simulink model "Satellite_Attitude_Control_Scenario_B_final"  (R2026a)
settings: Solver=ode23s  StopTime=100  MaxStep=1e-2
libraries: simulink x3, slpidlib x3, matrix_library x1
settings Model: Creator=sreecharan  LastModifiedBy=sreecharan

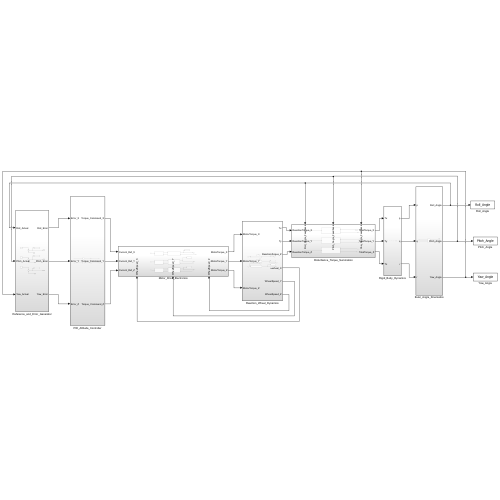
[thumbnail: Simulink's stored preview of the top-level diagram]
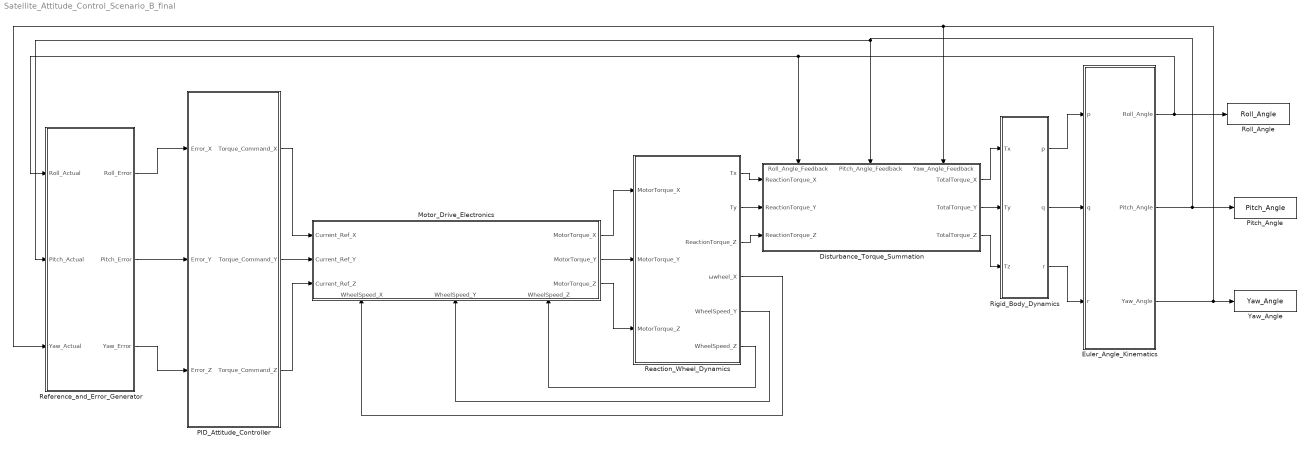
== system Satellite_Attitude_Control_Scenario_B_final ==
  Disturbance_Torque_Summation : Subsystem
      settings: PortSchema="{\"entries\":[{\"content\":{\"sides\":[{\"content\":{\"connectorIds\":[\"In1\",\"In2\",\"In3\"]},\"type\":\"ConnectorPlacement.EquallySpacedRectSide\",\"uuid\":\"7e4f6ff0-8d01-44c4-971d-6abc5d35a402\"},{\"content\":{\"connectorIds\":[\"Out1\",\"Out2\",\"Out3\"],\"side\":\"RIGHT\"},\"type\":\"ConnectorPlacement.EquallySpacedRectSide\",\"uuid\":\"cb81acf3-b383-4a7c-a155-f8d32ed2ffd6\"},{\"content\":{\"connectorIds\":[\"In4\",\"In5\",\"In6\"],\"side\":\"TOP\"},\"type\":\"ConnectorPlacement.EquallySpacedRectSide\",\"uuid\":\"aada53d5-02c2-40d2-a0ce-2f4cf8738fbf\"}]},\"type\":\"ConnectorPlacement.EquallySpacedConnector\",\"uuid\":\"ed5a9e7d-2126-4c89-bcb0-b7263c99b71f\"}],\"packageUris\":[\"http://schema.mathworks.com/mf0/Connector/R2020b\"],\"version\":\"1.0\"}"
  Euler_Angle_Kinematics : Subsystem
  Motor_Drive_Electronics : Subsystem
      settings: PortSchema="{\"entries\":[{\"content\":{\"sides\":[{\"content\":{\"connectorIds\":[\"In1\",\"In2\",\"In3\"]},\"type\":\"ConnectorPlacement.EquallySpacedRectSide\",\"uuid\":\"7e4f6ff0-8d01-44c4-971d-6abc5d35a402\"},{\"content\":{\"connectorIds\":[\"Out1\",\"Out2\",\"Out3\"],\"side\":\"RIGHT\"},\"type\":\"ConnectorPlacement.EquallySpacedRectSide\",\"uuid\":\"cb81acf3-b383-4a7c-a155-f8d32ed2ffd6\"},{\"content\":{\"side\":\"TOP\"},\"type\":\"ConnectorPlacement.EquallySpacedRectSide\",\"uuid\":\"aada53d5-02c2-40d2-a0ce-2f4cf8738fbf\"},{\"content\":{\"connectorIds\":[\"In4\",\"In5\",\"In6\"],\"side\":\"BOTTOM\"},\"type\":\"ConnectorPlacement.EquallySpacedRectSide\",\"uuid\":\"90859111-4cc3-4175-9d43-5206a627f844\"}]},\"type\":\"ConnectorPlacement.EquallySpacedConnector\",\"uuid\":\"ed5a9e7d-2126-4c89-bcb0-b7263c99b71f\"}],\"packageUris\":[\"http://schema.mathworks.com/mf0/Connector/R2020b\"],\"version\":\"1.0\"}"
  PID_Attitude_Controller : Subsystem
  Pitch_Angle : ToWorkspace  VariableName=Pitch_Angle  SampleTime=-1
  Reaction_Wheel_Dynamics : Subsystem
  Reference_and_Error_Generator : Subsystem
  Rigid_Body_Dynamics : Subsystem
  Roll_Angle : ToWorkspace  VariableName=Roll_Angle  SampleTime=-1
  Yaw_Angle : ToWorkspace  VariableName=Yaw_Angle  SampleTime=-1
  wires:
  Disturbance_Torque_Summation/1(TotalTorque_X) -> Rigid_Body_Dynamics/1(Tx)
  Disturbance_Torque_Summation/2(TotalTorque_Y) -> Rigid_Body_Dynamics/2(Ty)
  Disturbance_Torque_Summation/3(TotalTorque_Z) -> Rigid_Body_Dynamics/3(Tz)
  Motor_Drive_Electronics/2(MotorTorque_Y) -> Reaction_Wheel_Dynamics/2(MotorTorque_Y)
  Reaction_Wheel_Dynamics/1(Tx) -> Disturbance_Torque_Summation/1(ReactionTorque_X)
  Reaction_Wheel_Dynamics/2(Ty) -> Disturbance_Torque_Summation/2(ReactionTorque_Y)
  Reaction_Wheel_Dynamics/3(ReactionTorque_Z) -> Disturbance_Torque_Summation/3(ReactionTorque_Z)
  Reaction_Wheel_Dynamics/4(ωwheel_X) -> Motor_Drive_Electronics/4(WheelSpeed_X)
  Reaction_Wheel_Dynamics/5(WheelSpeed_Y) -> Motor_Drive_Electronics/5(WheelSpeed_Y)
  Reaction_Wheel_Dynamics/6(WheelSpeed_Z) -> Motor_Drive_Electronics/6(WheelSpeed_Z)
  Reference_and_Error_Generator/1(Roll_Error) -> PID_Attitude_Controller/1(Error_X)
  Reference_and_Error_Generator/2(Pitch_Error) -> PID_Attitude_Controller/2(Error_Y)
  Reference_and_Error_Generator/3(Yaw_Error) -> PID_Attitude_Controller/3(Error_Z)
  PID_Attitude_Controller/1(Torque_Command_X) -> Motor_Drive_Electronics/1(Current_Ref_X)
  PID_Attitude_Controller/2(Torque_Command_Y) -> Motor_Drive_Electronics/2(Current_Ref_Y)
  PID_Attitude_Controller/3(Torque_Command_Z) -> Motor_Drive_Electronics/3(Current_Ref_Z)
  Rigid_Body_Dynamics/1(p) -> Euler_Angle_Kinematics/1(p)
  Rigid_Body_Dynamics/2(q) -> Euler_Angle_Kinematics/2(q)
  Rigid_Body_Dynamics/3(r) -> Euler_Angle_Kinematics/3(r)
  Euler_Angle_Kinematics/1(Roll_Angle) -> Disturbance_Torque_Summation/4(Roll_Angle_Feedback), Reference_and_Error_Generator/1(Roll_Actual), Roll_Angle/1
  Euler_Angle_Kinematics/2(Pitch_Angle) -> Reference_and_Error_Generator/2(Pitch_Actual), Disturbance_Torque_Summation/5(Pitch_Angle_Feedback), Pitch_Angle/1
  Euler_Angle_Kinematics/3(Yaw_Angle) -> Disturbance_Torque_Summation/6(Yaw_Angle_Feedback), Reference_and_Error_Generator/3(Yaw_Actual), Yaw_Angle/1
  Motor_Drive_Electronics/3(MotorTorque_Z) -> Reaction_Wheel_Dynamics/3(MotorTorque_Z)
  Motor_Drive_Electronics/1(MotorTorque_X) -> Reaction_Wheel_Dynamics/1(MotorTorque_X)

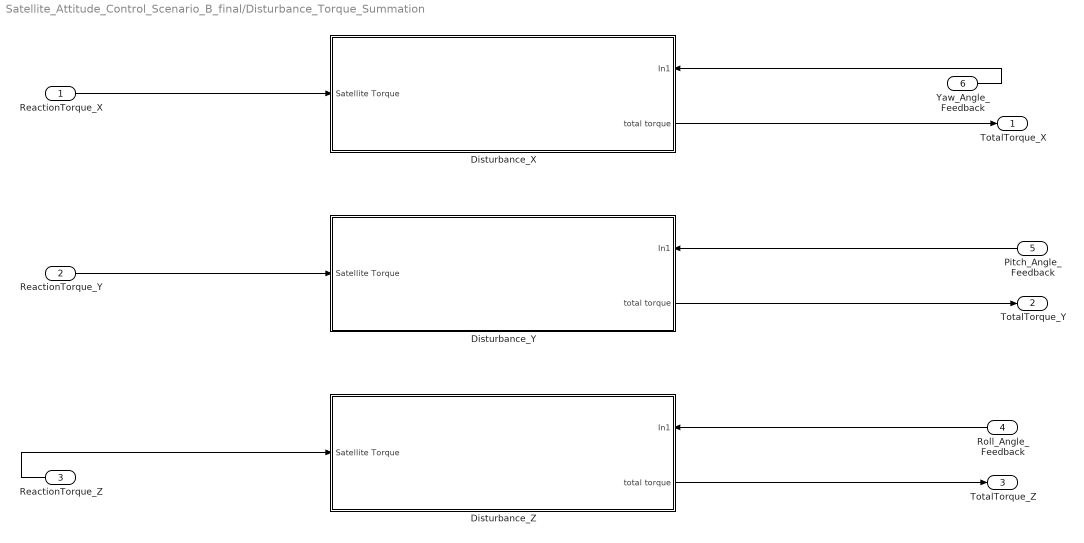
== system Satellite_Attitude_Control_Scenario_B_final/Disturbance_Torque_Summation ==
  ReactionTorque_X : Inport
  ReactionTorque_Y : Inport  Port=2
  ReactionTorque_Z : Inport  Port=3
  Roll_Angle_Feedback : Inport  Port=4
  Pitch_Angle_Feedback : Inport  Port=5
  Yaw_Angle_Feedback : Inport  Port=6
  Disturbance_X : Subsystem
      settings: PortSchema="{\"entries\":[{\"content\":{\"sides\":[{\"content\":{\"connectorIds\":[\"In1\"]},\"type\":\"ConnectorPlacement.EquallySpacedRectSide\",\"uuid\":\"e7f78c36-0d9a-4318-ba1f-4f96df5e40a9\"},{\"content\":{\"connectorIds\":[\"In2\",\"Out1\"],\"side\":\"RIGHT\"},\"type\":\"ConnectorPlacement.EquallySpacedRectSide\",\"uuid\":\"f98e017f-c554-4409-ad02-b03e27fbf9a0\"},{\"content\":{\"side\":\"TOP\"},\"type\":\"ConnectorPlacement.EquallySpacedRectSide\",\"uuid\":\"0f2d5841-4c85-457d-9c06-93d23c36a0cb\"}]},\"type\":\"ConnectorPlacement.EquallySpacedConnector\",\"uuid\":\"7906bc11-aae8-4996-900f-fb1686eb7203\"}],\"packageUris\":[\"http://schema.mathworks.com/mf0/Connector/R2020b\"],\"version\":\"1.0\"}"
  Disturbance_Y : Subsystem
      settings: PortSchema="{\"entries\":[{\"content\":{\"sides\":[{\"content\":{\"connectorIds\":[\"In1\"]},\"type\":\"ConnectorPlacement.EquallySpacedRectSide\",\"uuid\":\"e7f78c36-0d9a-4318-ba1f-4f96df5e40a9\"},{\"content\":{\"connectorIds\":[\"In2\",\"Out1\"],\"side\":\"RIGHT\"},\"type\":\"ConnectorPlacement.EquallySpacedRectSide\",\"uuid\":\"f98e017f-c554-4409-ad02-b03e27fbf9a0\"},{\"content\":{\"side\":\"TOP\"},\"type\":\"ConnectorPlacement.EquallySpacedRectSide\",\"uuid\":\"0f2d5841-4c85-457d-9c06-93d23c36a0cb\"}]},\"type\":\"ConnectorPlacement.EquallySpacedConnector\",\"uuid\":\"7906bc11-aae8-4996-900f-fb1686eb7203\"}],\"packageUris\":[\"http://schema.mathworks.com/mf0/Connector/R2020b\"],\"version\":\"1.0\"}"
  Disturbance_Z : Subsystem
      settings: PortSchema="{\"entries\":[{\"content\":{\"sides\":[{\"content\":{\"connectorIds\":[\"In1\"]},\"type\":\"ConnectorPlacement.EquallySpacedRectSide\",\"uuid\":\"e7f78c36-0d9a-4318-ba1f-4f96df5e40a9\"},{\"content\":{\"connectorIds\":[\"In2\",\"Out1\"],\"side\":\"RIGHT\"},\"type\":\"ConnectorPlacement.EquallySpacedRectSide\",\"uuid\":\"f98e017f-c554-4409-ad02-b03e27fbf9a0\"},{\"content\":{\"side\":\"TOP\"},\"type\":\"ConnectorPlacement.EquallySpacedRectSide\",\"uuid\":\"0f2d5841-4c85-457d-9c06-93d23c36a0cb\"}]},\"type\":\"ConnectorPlacement.EquallySpacedConnector\",\"uuid\":\"7906bc11-aae8-4996-900f-fb1686eb7203\"}],\"packageUris\":[\"http://schema.mathworks.com/mf0/Connector/R2020b\"],\"version\":\"1.0\"}"
  TotalTorque_X : Outport
  TotalTorque_Y : Outport  Port=2
  TotalTorque_Z : Outport  Port=3
  wires:
  Yaw_Angle_Feedback/1 -> Disturbance_X/2(In1)
  Disturbance_Z/1(total torque) -> TotalTorque_Z/1
  Disturbance_Y/1(total torque) -> TotalTorque_Y/1
  ReactionTorque_Y/1 -> Disturbance_Y/1(Satellite Torque)
  Roll_Angle_Feedback/1 -> Disturbance_Z/2(In1)
  Pitch_Angle_Feedback/1 -> Disturbance_Y/2(In1)
  ReactionTorque_Z/1 -> Disturbance_Z/1(Satellite Torque)
  Disturbance_X/1(total torque) -> TotalTorque_X/1
  ReactionTorque_X/1 -> Disturbance_X/1(Satellite Torque)

== system Satellite_Attitude_Control_Scenario_B_final/Euler_Angle_Kinematics ==
  p : Inport
  q : Inport  Port=2
  r : Inport  Port=3
  Euler Kinematics : Subsystem
  Roll_Angle : Outport
  Pitch_Angle : Outport  Port=2
  Yaw_Angle : Outport  Port=3
  wires:
  r/1 -> Euler Kinematics/3(r)
  Euler Kinematics/2(Pitch_Angle) -> Pitch_Angle/1
  Euler Kinematics/1(Roll_Angle) -> Roll_Angle/1
  p/1 -> Euler Kinematics/1(p)
  Euler Kinematics/3(Yaw_Angle) -> Yaw_Angle/1
  q/1 -> Euler Kinematics/2(q)

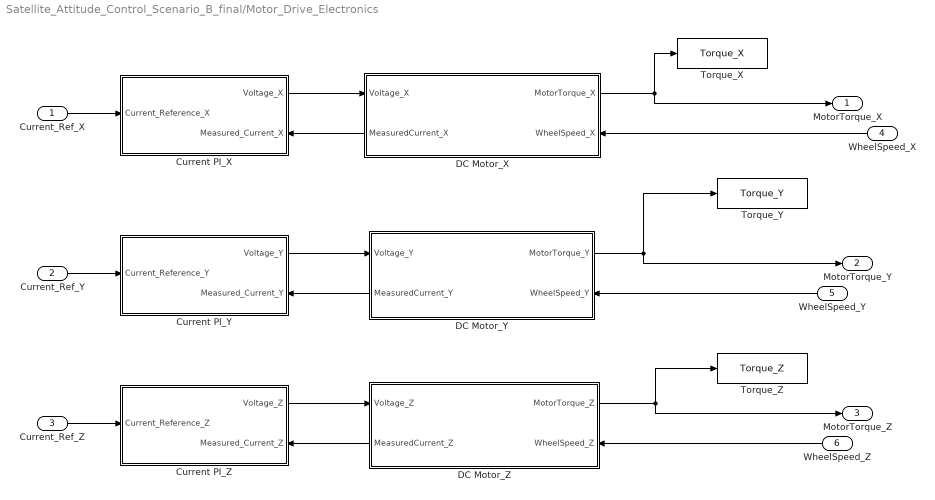
== system Satellite_Attitude_Control_Scenario_B_final/Motor_Drive_Electronics ==
  Current_Ref_X : Inport
  Current_Ref_Y : Inport  Port=2
  Current_Ref_Z : Inport  Port=3
  WheelSpeed_X : Inport  Port=4
  WheelSpeed_Y : Inport  Port=5
  WheelSpeed_Z : Inport  Port=6
  Current PI_X : Subsystem
      settings: PortSchema="{\"entries\":[{\"content\":{\"sides\":[{\"content\":{\"connectorIds\":[\"In1\"]},\"type\":\"ConnectorPlacement.EquallySpacedRectSide\",\"uuid\":\"ec13afe6-7a64-41e5-9104-27769ae66ec9\"},{\"content\":{\"connectorIds\":[\"Out1\",\"In2\"],\"side\":\"RIGHT\"},\"type\":\"ConnectorPlacement.EquallySpacedRectSide\",\"uuid\":\"7c3edc14-0315-4bf6-9ae7-ed8eab3e38cb\"},{\"content\":{\"side\":\"TOP\"},\"type\":\"ConnectorPlacement.EquallySpacedRectSide\",\"uuid\":\"2ff1a193-1271-4d3e-9081-11f4f33ce5f2\"}]},\"type\":\"ConnectorPlacement.EquallySpacedConnector\",\"uuid\":\"f73f2156-d72a-48d5-8aa2-510f5a049fc4\"}],\"packageUris\":[\"http://schema.mathworks.com/mf0/Connector/R2020b\"],\"version\":\"1.0\"}"
  Current PI_Y : Subsystem
      settings: PortSchema="{\"entries\":[{\"content\":{\"sides\":[{\"content\":{\"connectorIds\":[\"In1\"]},\"type\":\"ConnectorPlacement.EquallySpacedRectSide\",\"uuid\":\"ec13afe6-7a64-41e5-9104-27769ae66ec9\"},{\"content\":{\"connectorIds\":[\"Out1\",\"In2\"],\"side\":\"RIGHT\"},\"type\":\"ConnectorPlacement.EquallySpacedRectSide\",\"uuid\":\"7c3edc14-0315-4bf6-9ae7-ed8eab3e38cb\"},{\"content\":{\"side\":\"TOP\"},\"type\":\"ConnectorPlacement.EquallySpacedRectSide\",\"uuid\":\"2ff1a193-1271-4d3e-9081-11f4f33ce5f2\"}]},\"type\":\"ConnectorPlacement.EquallySpacedConnector\",\"uuid\":\"f73f2156-d72a-48d5-8aa2-510f5a049fc4\"}],\"packageUris\":[\"http://schema.mathworks.com/mf0/Connector/R2020b\"],\"version\":\"1.0\"}"
  Current PI_Z : Subsystem
      settings: PortSchema="{\"entries\":[{\"content\":{\"sides\":[{\"content\":{\"connectorIds\":[\"In1\"]},\"type\":\"ConnectorPlacement.EquallySpacedRectSide\",\"uuid\":\"ec13afe6-7a64-41e5-9104-27769ae66ec9\"},{\"content\":{\"connectorIds\":[\"Out1\",\"In2\"],\"side\":\"RIGHT\"},\"type\":\"ConnectorPlacement.EquallySpacedRectSide\",\"uuid\":\"7c3edc14-0315-4bf6-9ae7-ed8eab3e38cb\"},{\"content\":{\"side\":\"TOP\"},\"type\":\"ConnectorPlacement.EquallySpacedRectSide\",\"uuid\":\"2ff1a193-1271-4d3e-9081-11f4f33ce5f2\"}]},\"type\":\"ConnectorPlacement.EquallySpacedConnector\",\"uuid\":\"f73f2156-d72a-48d5-8aa2-510f5a049fc4\"}],\"packageUris\":[\"http://schema.mathworks.com/mf0/Connector/R2020b\"],\"version\":\"1.0\"}"
  DC Motor_X : Subsystem
      settings: PortSchema="{\"entries\":[{\"content\":{\"sides\":[{\"content\":{\"connectorIds\":[\"In1\",\"Out2\"]},\"type\":\"ConnectorPlacement.EquallySpacedRectSide\",\"uuid\":\"6decb560-04e7-4e3c-a8d2-82b3e040f40c\"},{\"content\":{\"connectorIds\":[\"Out1\",\"In2\"],\"side\":\"RIGHT\"},\"type\":\"ConnectorPlacement.EquallySpacedRectSide\",\"uuid\":\"b717ceb4-825a-4dcd-8046-00b2b9fe843a\"},{\"content\":{\"side\":\"TOP\"},\"type\":\"ConnectorPlacement.EquallySpacedRectSide\",\"uuid\":\"a28e7354-c407-42ac-a7f5-63ca03116f72\"}]},\"type\":\"ConnectorPlacement.EquallySpacedConnector\",\"uuid\":\"b0d58d04-64b3-4ef6-b545-4c8a298f2fb2\"}],\"packageUris\":[\"http://schema.mathworks.com/mf0/Connector/R2020b\"],\"version\":\"1.0\"}"
  DC Motor_Y : Subsystem
      settings: PortSchema="{\"entries\":[{\"content\":{\"sides\":[{\"content\":{\"connectorIds\":[\"In1\",\"Out2\"]},\"type\":\"ConnectorPlacement.EquallySpacedRectSide\",\"uuid\":\"6decb560-04e7-4e3c-a8d2-82b3e040f40c\"},{\"content\":{\"connectorIds\":[\"Out1\",\"In2\"],\"side\":\"RIGHT\"},\"type\":\"ConnectorPlacement.EquallySpacedRectSide\",\"uuid\":\"b717ceb4-825a-4dcd-8046-00b2b9fe843a\"},{\"content\":{\"side\":\"TOP\"},\"type\":\"ConnectorPlacement.EquallySpacedRectSide\",\"uuid\":\"a28e7354-c407-42ac-a7f5-63ca03116f72\"}]},\"type\":\"ConnectorPlacement.EquallySpacedConnector\",\"uuid\":\"b0d58d04-64b3-4ef6-b545-4c8a298f2fb2\"}],\"packageUris\":[\"http://schema.mathworks.com/mf0/Connector/R2020b\"],\"version\":\"1.0\"}"
  DC Motor_Z : Subsystem
      settings: PortSchema="{\"entries\":[{\"content\":{\"sides\":[{\"content\":{\"connectorIds\":[\"In1\",\"Out2\"]},\"type\":\"ConnectorPlacement.EquallySpacedRectSide\",\"uuid\":\"6decb560-04e7-4e3c-a8d2-82b3e040f40c\"},{\"content\":{\"connectorIds\":[\"Out1\",\"In2\"],\"side\":\"RIGHT\"},\"type\":\"ConnectorPlacement.EquallySpacedRectSide\",\"uuid\":\"b717ceb4-825a-4dcd-8046-00b2b9fe843a\"},{\"content\":{\"side\":\"TOP\"},\"type\":\"ConnectorPlacement.EquallySpacedRectSide\",\"uuid\":\"a28e7354-c407-42ac-a7f5-63ca03116f72\"}]},\"type\":\"ConnectorPlacement.EquallySpacedConnector\",\"uuid\":\"b0d58d04-64b3-4ef6-b545-4c8a298f2fb2\"}],\"packageUris\":[\"http://schema.mathworks.com/mf0/Connector/R2020b\"],\"version\":\"1.0\"}"
  Torque_X : ToWorkspace  VariableName=Torque_X  SampleTime=-1
  Torque_Y : ToWorkspace  VariableName=Torque_Y  SampleTime=-1
  Torque_Z : ToWorkspace  VariableName=Torque_Z  SampleTime=-1
  MotorTorque_X : Outport
  MotorTorque_Y : Outport  Port=2
  MotorTorque_Z : Outport  Port=3
  wires:
  Current PI_Z/1(Voltage_Z) -> DC Motor_Z/1(Voltage_Z)
  DC Motor_X/2(MeasuredCurrent_X) -> Current PI_X/2(Measured_Current_X)
  DC Motor_Y/1(MotorTorque_Y) -> MotorTorque_Y/1, Torque_Y/1
  DC Motor_X/1(MotorTorque_X) -> MotorTorque_X/1, Torque_X/1
  DC Motor_Z/2(MeasuredCurrent_Z) -> Current PI_Z/2(Measured_Current_Z)
  DC Motor_Y/2(MeasuredCurrent_Y) -> Current PI_Y/2(Measured_Current_Y)
  DC Motor_Z/1(MotorTorque_Z) -> MotorTorque_Z/1, Torque_Z/1
  Current PI_Y/1(Voltage_Y) -> DC Motor_Y/1(Voltage_Y)
  Current PI_X/1(Voltage_X) -> DC Motor_X/1(Voltage_X)
  Current_Ref_Z/1 -> Current PI_Z/1(Current_Reference_Z)
  Current_Ref_Y/1 -> Current PI_Y/1(Current_Reference_Y)
  WheelSpeed_X/1 -> DC Motor_X/2(WheelSpeed_X)
  WheelSpeed_Y/1 -> DC Motor_Y/2(WheelSpeed_Y)
  Current_Ref_X/1 -> Current PI_X/1(Current_Reference_X)
  WheelSpeed_Z/1 -> DC Motor_Z/2(WheelSpeed_Z)

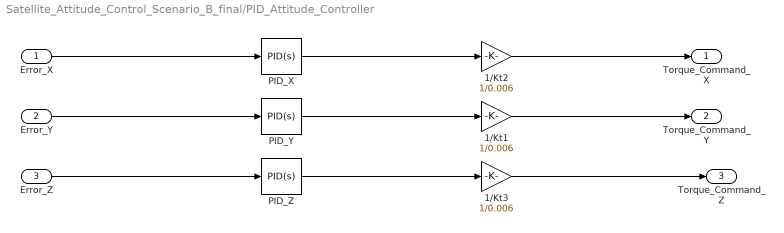
== system Satellite_Attitude_Control_Scenario_B_final/PID_Attitude_Controller ==
  Error_X : Inport
  Error_Y : Inport  Port=2
  Error_Z : Inport  Port=3
  1/Kt1 : Gain  Gain=1/0.006
  1/Kt2 : Gain  Gain=1/0.006
  1/Kt3 : Gain  Gain=1/0.006
  PID_X : slpidlib/PID Controller  Controller=PID  Form=Parallel  TimeDomain=Continuous-time  UseExternalTs=off  SampleTime=-1  IntegratorMethod=Forward Euler  FilterMethod=Forward Euler  ControllerParametersSource=internal  P=0.015  I=0.002  UseKiTs=off  D=0.045  UseExternalDerivativeSource=off  N=100  UseFilter=on  TunerSelectOption=Transfer Function Based (PID Tuner App)  InitialConditionSource=internal  InitialConditionForIntegrator=0  InitialConditionForFilter=0  DifferentiatorICPrevScaledInput=0  ExternalReset=none  TrackingMode=off  Kt=1  LimitOutput=on  SatLimitsSource=internal  UpperSaturationLimit=0.008  LowerSaturationLimit=-0.008  LinearizeAsGain=on  AntiWindupMode=none  Kb=1  LimitIntegrator=off  UpperIntegratorSaturationLimit=inf  LowerIntegratorSaturationLimit=-inf  POutMin=[]  POutMax=[]  IOutMin=[]  IOutMax=[]  DOutMin=[]  DOutMax=[]  NOutMin=[]  NOutMax=[]  SumOutMin=[]  SumOutMax=[]  SaturationOutMin=[]  SaturationOutMax=[]  PParamMin=[]  PParamMax=[]  IParamMin=[]  IParamMax=[]  DParamMin=[]  DParamMax=[]  NParamMin=[]  NParamMax=[]  KbParamMin=[]  KbParamMax=[]  KtParamMin=[]  KtParamMax=[]  KbOutMin=[]  KbOutMax=[]  KtOutMin=[]  KtOutMax=[]  IntegratorOutMin=[]  IntegratorOutMax=[]  FilterOutMin=[]  FilterOutMax=[]  SumI1OutMin=[]  SumI1OutMax=[]  SumI2OutMin=[]  SumI2OutMax=[]  SumI3OutMin=[]  SumI3OutMax=[]  SumI4OutMin=[]  SumI4OutMax=[]  SumDOutMin=[]  SumDOutMax=[]  DifferentiatorOutMin=[]  DifferentiatorOutMax=[]  FilterDiffOutCoefMin=[]  FilterDiffOutCoefMax=[]  ReciprocalOutMin=[]  ReciprocalOutMax=[]  SumDenOutMin=[]  SumDenOutMax=[]  SumNumOutMin=[]  SumNumOutMax=[]  DivideOutMin=[]  DivideOutMax=[]  UdiffTsProdOutMin=[]  UdiffTsProdOutMax=[]  NTsProdOutMin=[]  NTsProdOutMax=[]  UintegralTsProdOutMin=[]  UintegralTsProdOutMax=[]  UngainTsProdOutMin=[]  UngainTsProdOutMax=[]  ClampingZeroOutDataTypeStr=Inherit: Inherit via back propagation  ClampingZeroOutMin=[]  ClampingZeroOutMax=[]  FilterDenConstantOutDataTypeStr=Inherit: Inherit via back propagation  FilterDenConstantOutMin=[]  FilterDenConstantOutMax=[]  PCopyOutDataTypeStr=Inherit: Inherit via back propagation  PCopyOutMin=[]  PCopyOutMax=[]  NCopyOutDataTypeStr=Inherit: Inherit via back propagation  NCopyOutMin=[]  NCopyOutMax=[]  IntegratorContinuousStateAttributes=''  IntegratorStateMustResolveToSignalObject=off  IntegratorRTWStateStorageClass=Auto  FilterContinuousStateAttributes=''  FilterStateMustResolveToSignalObject=off  FilterRTWStateStorageClass=Auto  ParallelPVariant=InternalParameters  IdealPVariant=Disabled  IVariant=InternalParameters  DVariant=InternalParameters  IntegratorVariant=Continuous  SatVariant=Enabled  AWVariant=Passthrough  PCopyVariant=Disabled  TRVariant=Disabled  FdbkBlocksVariant=Forward  IdealPFdbkVariant=Disabled  SatFdbkVariant=Disabled  DerivativeFilterVariant=ContFilter  NVariant=InternalParameters  NCopyVariant=Disabled  FilterICVariant=InternalICsFilter  IntegratorICVariant=InternalICs  ExternalResetVariant=Disabled  TRSumVariant=Passthrough  SumFdbkVariant=Disabled  SumVariant=Sum_PID  TsampFilterVariant=InternalTs  TsampNgainVariant=Passthrough  TsampIntegralVariant=Disabled_SignalSpec  ExternalSaturationOutDataTypeStr=Inherit: Same as second input  DerivativeSourceVariant=ErrorSignal  PreIntVariant=InternalPreInt
  PID_Y : slpidlib/PID Controller  Controller=PID  Form=Parallel  TimeDomain=Continuous-time  UseExternalTs=off  SampleTime=-1  IntegratorMethod=Forward Euler  FilterMethod=Forward Euler  ControllerParametersSource=internal  P=0.0544  I=0.0061  UseKiTs=off  D=0.05  UseExternalDerivativeSource=off  N=100  UseFilter=on  TunerSelectOption=Transfer Function Based (PID Tuner App)  InitialConditionSource=internal  InitialConditionForIntegrator=0  InitialConditionForFilter=0  DifferentiatorICPrevScaledInput=0  ExternalReset=none  TrackingMode=off  Kt=1  LimitOutput=on  SatLimitsSource=internal  UpperSaturationLimit=0.008  LowerSaturationLimit=-0.008  LinearizeAsGain=on  AntiWindupMode=none  Kb=1  LimitIntegrator=off  UpperIntegratorSaturationLimit=inf  LowerIntegratorSaturationLimit=-inf  POutMin=[]  POutMax=[]  IOutMin=[]  IOutMax=[]  DOutMin=[]  DOutMax=[]  NOutMin=[]  NOutMax=[]  SumOutMin=[]  SumOutMax=[]  SaturationOutMin=[]  SaturationOutMax=[]  PParamMin=[]  PParamMax=[]  IParamMin=[]  IParamMax=[]  DParamMin=[]  DParamMax=[]  NParamMin=[]  NParamMax=[]  KbParamMin=[]  KbParamMax=[]  KtParamMin=[]  KtParamMax=[]  KbOutMin=[]  KbOutMax=[]  KtOutMin=[]  KtOutMax=[]  IntegratorOutMin=[]  IntegratorOutMax=[]  FilterOutMin=[]  FilterOutMax=[]  SumI1OutMin=[]  SumI1OutMax=[]  SumI2OutMin=[]  SumI2OutMax=[]  SumI3OutMin=[]  SumI3OutMax=[]  SumI4OutMin=[]  SumI4OutMax=[]  SumDOutMin=[]  SumDOutMax=[]  DifferentiatorOutMin=[]  DifferentiatorOutMax=[]  FilterDiffOutCoefMin=[]  FilterDiffOutCoefMax=[]  ReciprocalOutMin=[]  ReciprocalOutMax=[]  SumDenOutMin=[]  SumDenOutMax=[]  SumNumOutMin=[]  SumNumOutMax=[]  DivideOutMin=[]  DivideOutMax=[]  UdiffTsProdOutMin=[]  UdiffTsProdOutMax=[]  NTsProdOutMin=[]  NTsProdOutMax=[]  UintegralTsProdOutMin=[]  UintegralTsProdOutMax=[]  UngainTsProdOutMin=[]  UngainTsProdOutMax=[]  ClampingZeroOutDataTypeStr=Inherit: Inherit via back propagation  ClampingZeroOutMin=[]  ClampingZeroOutMax=[]  FilterDenConstantOutDataTypeStr=Inherit: Inherit via back propagation  FilterDenConstantOutMin=[]  FilterDenConstantOutMax=[]  PCopyOutDataTypeStr=Inherit: Inherit via back propagation  PCopyOutMin=[]  PCopyOutMax=[]  NCopyOutDataTypeStr=Inherit: Inherit via back propagation  NCopyOutMin=[]  NCopyOutMax=[]  IntegratorContinuousStateAttributes=''  IntegratorStateMustResolveToSignalObject=off  IntegratorRTWStateStorageClass=Auto  FilterContinuousStateAttributes=''  FilterStateMustResolveToSignalObject=off  FilterRTWStateStorageClass=Auto  ParallelPVariant=InternalParameters  IdealPVariant=Disabled  IVariant=InternalParameters  DVariant=InternalParameters  IntegratorVariant=Continuous  SatVariant=Enabled  AWVariant=Passthrough  PCopyVariant=Disabled  TRVariant=Disabled  FdbkBlocksVariant=Forward  IdealPFdbkVariant=Disabled  SatFdbkVariant=Disabled  DerivativeFilterVariant=ContFilter  NVariant=InternalParameters  NCopyVariant=Disabled  FilterICVariant=InternalICsFilter  IntegratorICVariant=InternalICs  ExternalResetVariant=Disabled  TRSumVariant=Passthrough  SumFdbkVariant=Disabled  SumVariant=Sum_PID  TsampFilterVariant=InternalTs  TsampNgainVariant=Passthrough  TsampIntegralVariant=Disabled_SignalSpec  ExternalSaturationOutDataTypeStr=Inherit: Same as second input  DerivativeSourceVariant=ErrorSignal  PreIntVariant=InternalPreInt
  PID_Z : slpidlib/PID Controller  Controller=PID  Form=Parallel  TimeDomain=Continuous-time  UseExternalTs=off  SampleTime=-1  IntegratorMethod=Forward Euler  FilterMethod=Forward Euler  ControllerParametersSource=internal  P=0.015  I=0.002  UseKiTs=off  D=0.045  UseExternalDerivativeSource=off  N=100  UseFilter=on  TunerSelectOption=Transfer Function Based (PID Tuner App)  InitialConditionSource=internal  InitialConditionForIntegrator=0  InitialConditionForFilter=0  DifferentiatorICPrevScaledInput=0  ExternalReset=none  TrackingMode=off  Kt=1  LimitOutput=on  SatLimitsSource=internal  UpperSaturationLimit=0.008  LowerSaturationLimit=-0.008  LinearizeAsGain=on  AntiWindupMode=none  Kb=1  LimitIntegrator=on  UpperIntegratorSaturationLimit=inf  LowerIntegratorSaturationLimit=-inf  POutMin=[]  POutMax=[]  IOutMin=[]  IOutMax=[]  DOutMin=[]  DOutMax=[]  NOutMin=[]  NOutMax=[]  SumOutMin=[]  SumOutMax=[]  SaturationOutMin=[]  SaturationOutMax=[]  PParamMin=[]  PParamMax=[]  IParamMin=[]  IParamMax=[]  DParamMin=[]  DParamMax=[]  NParamMin=[]  NParamMax=[]  KbParamMin=[]  KbParamMax=[]  KtParamMin=[]  KtParamMax=[]  KbOutMin=[]  KbOutMax=[]  KtOutMin=[]  KtOutMax=[]  IntegratorOutMin=[]  IntegratorOutMax=[]  FilterOutMin=[]  FilterOutMax=[]  SumI1OutMin=[]  SumI1OutMax=[]  SumI2OutMin=[]  SumI2OutMax=[]  SumI3OutMin=[]  SumI3OutMax=[]  SumI4OutMin=[]  SumI4OutMax=[]  SumDOutMin=[]  SumDOutMax=[]  DifferentiatorOutMin=[]  DifferentiatorOutMax=[]  FilterDiffOutCoefMin=[]  FilterDiffOutCoefMax=[]  ReciprocalOutMin=[]  ReciprocalOutMax=[]  SumDenOutMin=[]  SumDenOutMax=[]  SumNumOutMin=[]  SumNumOutMax=[]  DivideOutMin=[]  DivideOutMax=[]  UdiffTsProdOutMin=[]  UdiffTsProdOutMax=[]  NTsProdOutMin=[]  NTsProdOutMax=[]  UintegralTsProdOutMin=[]  UintegralTsProdOutMax=[]  UngainTsProdOutMin=[]  UngainTsProdOutMax=[]  ClampingZeroOutDataTypeStr=Inherit: Inherit via back propagation  ClampingZeroOutMin=[]  ClampingZeroOutMax=[]  FilterDenConstantOutDataTypeStr=Inherit: Inherit via back propagation  FilterDenConstantOutMin=[]  FilterDenConstantOutMax=[]  PCopyOutDataTypeStr=Inherit: Inherit via back propagation  PCopyOutMin=[]  PCopyOutMax=[]  NCopyOutDataTypeStr=Inherit: Inherit via back propagation  NCopyOutMin=[]  NCopyOutMax=[]  IntegratorContinuousStateAttributes=''  IntegratorStateMustResolveToSignalObject=off  IntegratorRTWStateStorageClass=Auto  FilterContinuousStateAttributes=''  FilterStateMustResolveToSignalObject=off  FilterRTWStateStorageClass=Auto  ParallelPVariant=InternalParameters  IdealPVariant=Disabled  IVariant=InternalParameters  DVariant=InternalParameters  IntegratorVariant=Continuous  SatVariant=Enabled  AWVariant=Passthrough  PCopyVariant=Disabled  TRVariant=Disabled  FdbkBlocksVariant=Forward  IdealPFdbkVariant=Disabled  SatFdbkVariant=Disabled  DerivativeFilterVariant=ContFilter  NVariant=InternalParameters  NCopyVariant=Disabled  FilterICVariant=InternalICsFilter  IntegratorICVariant=InternalICs  ExternalResetVariant=Disabled  TRSumVariant=Passthrough  SumFdbkVariant=Disabled  SumVariant=Sum_PID  TsampFilterVariant=InternalTs  TsampNgainVariant=Passthrough  TsampIntegralVariant=Disabled_SignalSpec  ExternalSaturationOutDataTypeStr=Inherit: Same as second input  DerivativeSourceVariant=ErrorSignal  PreIntVariant=InternalPreInt
  Torque_Command_X : Outport
  Torque_Command_Y : Outport  Port=2
  Torque_Command_Z : Outport  Port=3
  wires:
  PID_Z/1 -> 1/Kt3/1
  1/Kt2/1 -> Torque_Command_X/1
  1/Kt3/1 -> Torque_Command_Z/1
  Error_Y/1 -> PID_Y/1
  PID_Y/1 -> 1/Kt1/1
  PID_X/1 -> 1/Kt2/1
  1/Kt1/1 -> Torque_Command_Y/1
  Error_Z/1 -> PID_Z/1
  Error_X/1 -> PID_X/1

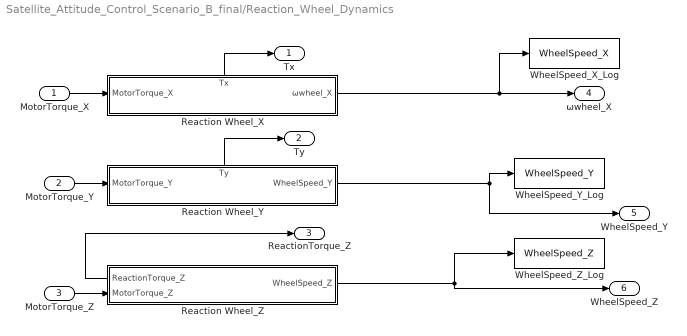
== system Satellite_Attitude_Control_Scenario_B_final/Reaction_Wheel_Dynamics ==
  MotorTorque_X : Inport
  MotorTorque_Y : Inport  Port=2
  MotorTorque_Z : Inport  Port=3
  Reaction Wheel_X : Subsystem
      settings: PortSchema="{\"entries\":[{\"content\":{\"sides\":[{\"content\":{\"connectorIds\":[\"In1\"]},\"type\":\"ConnectorPlacement.EquallySpacedRectSide\",\"uuid\":\"5dbcf71b-4bbb-463b-beea-80ab16e1a559\"},{\"content\":{\"connectorIds\":[\"Out1\"],\"side\":\"RIGHT\"},\"type\":\"ConnectorPlacement.EquallySpacedRectSide\",\"uuid\":\"2ea40819-5353-4131-8956-55917f52d00c\"},{\"content\":{\"connectorIds\":[\"Out2\"],\"side\":\"TOP\"},\"type\":\"ConnectorPlacement.EquallySpacedRectSide\",\"uuid\":\"c59e7123-e0d0-45cb-aaed-c6c85372aea0\"}]},\"type\":\"ConnectorPlacement.EquallySpacedConnector\",\"uuid\":\"1d5021f4-2059-4a45-8503-4e7cffae7b0a\"}],\"packageUris\":[\"http://schema.mathworks.com/mf0/Connector/R2020b\"],\"version\":\"1.0\"}"
  Reaction Wheel_Y : Subsystem
      settings: PortSchema="{\"entries\":[{\"content\":{\"sides\":[{\"content\":{\"connectorIds\":[\"In1\"]},\"type\":\"ConnectorPlacement.EquallySpacedRectSide\",\"uuid\":\"5dbcf71b-4bbb-463b-beea-80ab16e1a559\"},{\"content\":{\"connectorIds\":[\"Out1\"],\"side\":\"RIGHT\"},\"type\":\"ConnectorPlacement.EquallySpacedRectSide\",\"uuid\":\"2ea40819-5353-4131-8956-55917f52d00c\"},{\"content\":{\"connectorIds\":[\"Out2\"],\"side\":\"TOP\"},\"type\":\"ConnectorPlacement.EquallySpacedRectSide\",\"uuid\":\"c59e7123-e0d0-45cb-aaed-c6c85372aea0\"}]},\"type\":\"ConnectorPlacement.EquallySpacedConnector\",\"uuid\":\"1d5021f4-2059-4a45-8503-4e7cffae7b0a\"}],\"packageUris\":[\"http://schema.mathworks.com/mf0/Connector/R2020b\"],\"version\":\"1.0\"}"
  Reaction Wheel_Z : Subsystem
      settings: PortSchema="{\"entries\":[{\"content\":{\"sides\":[{\"content\":{\"connectorIds\":[\"Out2\",\"In1\"]},\"type\":\"ConnectorPlacement.EquallySpacedRectSide\",\"uuid\":\"5dbcf71b-4bbb-463b-beea-80ab16e1a559\"},{\"content\":{\"connectorIds\":[\"Out1\"],\"side\":\"RIGHT\"},\"type\":\"ConnectorPlacement.EquallySpacedRectSide\",\"uuid\":\"2ea40819-5353-4131-8956-55917f52d00c\"},{\"content\":{\"side\":\"TOP\"},\"type\":\"ConnectorPlacement.EquallySpacedRectSide\",\"uuid\":\"c59e7123-e0d0-45cb-aaed-c6c85372aea0\"}]},\"type\":\"ConnectorPlacement.EquallySpacedConnector\",\"uuid\":\"1d5021f4-2059-4a45-8503-4e7cffae7b0a\"}],\"packageUris\":[\"http://schema.mathworks.com/mf0/Connector/R2020b\"],\"version\":\"1.0\"}"
  WheelSpeed_X_Log : ToWorkspace  VariableName=WheelSpeed_X  SampleTime=-1
  WheelSpeed_Y_Log : ToWorkspace  VariableName=WheelSpeed_Y  SampleTime=-1
  WheelSpeed_Z_Log : ToWorkspace  VariableName=WheelSpeed_Z  SampleTime=-1
  Tx : Outport
  Ty : Outport  Port=2
  ReactionTorque_Z : Outport  Port=3
  ωwheel_X : Outport  Port=4
  WheelSpeed_Y : Outport  Port=5
  WheelSpeed_Z : Outport  Port=6
  wires:
  Reaction Wheel_Y/1(WheelSpeed_Y) -> WheelSpeed_Y/1, WheelSpeed_Y_Log/1
  Reaction Wheel_X/1(ωwheel_X) -> ωwheel_X/1, WheelSpeed_X_Log/1
  MotorTorque_X/1 -> Reaction Wheel_X/1(MotorTorque_X)
  Reaction Wheel_Z/1(WheelSpeed_Z) -> WheelSpeed_Z/1, WheelSpeed_Z_Log/1
  Reaction Wheel_Z/2(ReactionTorque_Z) -> ReactionTorque_Z/1
  MotorTorque_Y/1 -> Reaction Wheel_Y/1(MotorTorque_Y)
  MotorTorque_Z/1 -> Reaction Wheel_Z/1(MotorTorque_Z)
  Reaction Wheel_X/2(Tx) -> Tx/1
  Reaction Wheel_Y/2(Ty) -> Ty/1

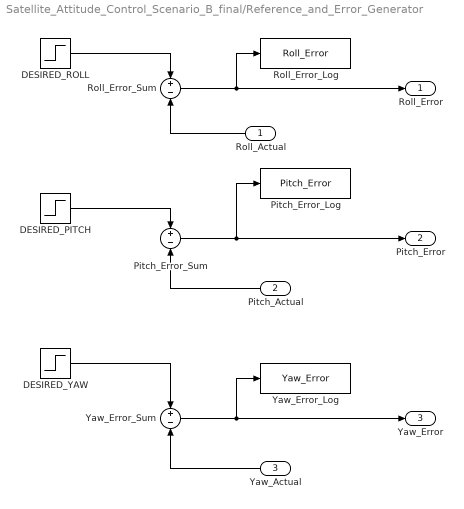
== system Satellite_Attitude_Control_Scenario_B_final/Reference_and_Error_Generator ==
  Roll_Actual : Inport
  Pitch_Actual : Inport  Port=2
  Yaw_Actual : Inport  Port=3
  DESIRED_PITCH : Step  FinalValue=pi/6  SampleTime=0
  DESIRED_ROLL : Step  FinalValue=pi/3  SampleTime=0
  DESIRED_YAW : Step  FinalValue=pi/4  SampleTime=0
  Pitch_Error_Log : ToWorkspace  VariableName=Pitch_Error  SampleTime=-1
  Pitch_Error_Sum : Sum  Inputs=+-
  Roll_Error_Log : ToWorkspace  VariableName=Roll_Error  SampleTime=-1
  Roll_Error_Sum : Sum  Inputs=+-
  Yaw_Error_Log : ToWorkspace  VariableName=Yaw_Error  SampleTime=-1
  Yaw_Error_Sum : Sum  Inputs=+-
  Roll_Error : Outport
  Pitch_Error : Outport  Port=2
  Yaw_Error : Outport  Port=3
  wires:
  DESIRED_ROLL/1 -> Roll_Error_Sum/1
  Yaw_Error_Sum/1 -> Yaw_Error/1, Yaw_Error_Log/1
  DESIRED_PITCH/1 -> Pitch_Error_Sum/1
  Roll_Error_Sum/1 -> Roll_Error/1, Roll_Error_Log/1
  Pitch_Error_Sum/1 -> Pitch_Error/1, Pitch_Error_Log/1
  DESIRED_YAW/1 -> Yaw_Error_Sum/1
  Yaw_Actual/1 -> Yaw_Error_Sum/2
  Roll_Actual/1 -> Roll_Error_Sum/2
  Pitch_Actual/1 -> Pitch_Error_Sum/2

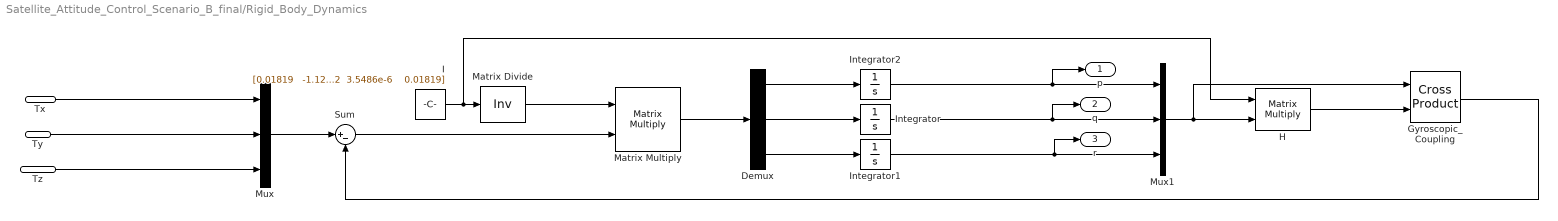
== system Satellite_Attitude_Control_Scenario_B_final/Rigid_Body_Dynamics ==
  Tx : Inport
  Ty : Inport  Port=2
  Tz : Inport  Port=3
  Demux : Demux  Outputs=3
  Gyroscopic_Coupling : matrix_library/Cross Product
  H : Product  Multiplication=Matrix(*)
  I : Constant  Value=|  VectorParams1D=off
      | [0.01819   -1.1289e-5   -0.005382;
      |  -1.1289e-5 0.01238      3.5486e-6;
      |  -0.005382  3.5486e-6    0.01819]
  Integrator : Integrator
  Integrator1 : Integrator
  Integrator2 : Integrator
  Matrix Divide : Product  Inputs=/  Multiplication=Matrix(*)
  Matrix Multiply : Product  Multiplication=Matrix(*)
  Mux : Mux  Inputs=3
  Mux1 : Mux  Inputs=3
  Sum : Sum  Inputs=|+-
  p : Outport
  q : Outport  Port=2
  r : Outport  Port=3
  wires:
  Tx/1 -> Mux/1
  Ty/1 -> Mux/2
  Tz/1 -> Mux/3
  H/1 -> Gyroscopic_Coupling/2
  Gyroscopic_Coupling/1 -> Sum/2
  Mux/1 -> Sum/1
  Matrix Divide/1 -> Matrix Multiply/1
  Sum/1 -> Matrix Multiply/2
  Matrix Multiply/1 -> Demux/1
  Demux/1 -> Integrator2/1
  Demux/2 -> Integrator/1
  Demux/3 -> Integrator1/1
  Integrator1/1 -> r/1, Mux1/3
  Integrator/1 -> q/1, Mux1/2
  Integrator2/1 -> p/1, Mux1/1
  Mux1/1 -> Gyroscopic_Coupling/1, H/2
  I/1 -> H/1, Matrix Divide/1

== system Satellite_Attitude_Control_Scenario_B_final/Disturbance_Torque_Summation/Disturbance_X ==
  Satellite Torque : Inport
  In1 : Inport  Port=2
  Aerodynamic Drag : Subsystem
  Constant disturbance : Constant  Value=1e-7
  Gravity-Gradient : Subsystem
  Solar Radiation Pressure : Subsystem
  Sum : Sum  Inputs=|++++++
  White Noise : Subsystem
  total torque : Outport
  wires:
  In1/1 -> Gravity-Gradient/1(Theta)
  Aerodynamic Drag/1(Out1) -> Sum/3
  Solar Radiation Pressure/1(Out1) -> Sum/4
  White Noise/1(Out1) -> Sum/5
  Constant disturbance/1 -> Sum/6
  Gravity-Gradient/1(Tdist) -> Sum/2
  Sum/1 -> total torque/1
  Satellite Torque/1 -> Sum/1

== system Satellite_Attitude_Control_Scenario_B_final/Disturbance_Torque_Summation/Disturbance_Y ==
  Satellite Torque : Inport
  In1 : Inport  Port=2
  Aerodynamic Drag : Subsystem
  Constant disturbance : Constant  Value=3e-7
  Gravity-Gradient : Subsystem
  Solar Radiation Pressure : Subsystem
  Sum : Sum  Inputs=|++++++
  White Noise : Subsystem
  total torque : Outport
  wires:
  In1/1 -> Gravity-Gradient/1(Theta)
  Aerodynamic Drag/1(Out1) -> Sum/3
  Solar Radiation Pressure/1(Out1) -> Sum/4
  White Noise/1(Out1) -> Sum/5
  Constant disturbance/1 -> Sum/6
  Gravity-Gradient/1(Tdist) -> Sum/2
  Sum/1 -> total torque/1
  Satellite Torque/1 -> Sum/1

== system Satellite_Attitude_Control_Scenario_B_final/Disturbance_Torque_Summation/Disturbance_Z ==
  Satellite Torque : Inport
  In1 : Inport  Port=2
  Aerodynamic Drag : Subsystem
  Constant disturbance : Constant  Value=2e-7
  Gravity-Gradient : Subsystem
  Solar Radiation Pressure : Subsystem
  Sum : Sum  Inputs=|++++++
  White Noise : Subsystem
  total torque : Outport
  wires:
  In1/1 -> Gravity-Gradient/1(Theta)
  Aerodynamic Drag/1(Out1) -> Sum/3
  Solar Radiation Pressure/1(Out1) -> Sum/4
  White Noise/1(Out1) -> Sum/5
  Constant disturbance/1 -> Sum/6
  Gravity-Gradient/1(Tdist) -> Sum/2
  Sum/1 -> total torque/1
  Satellite Torque/1 -> Sum/1

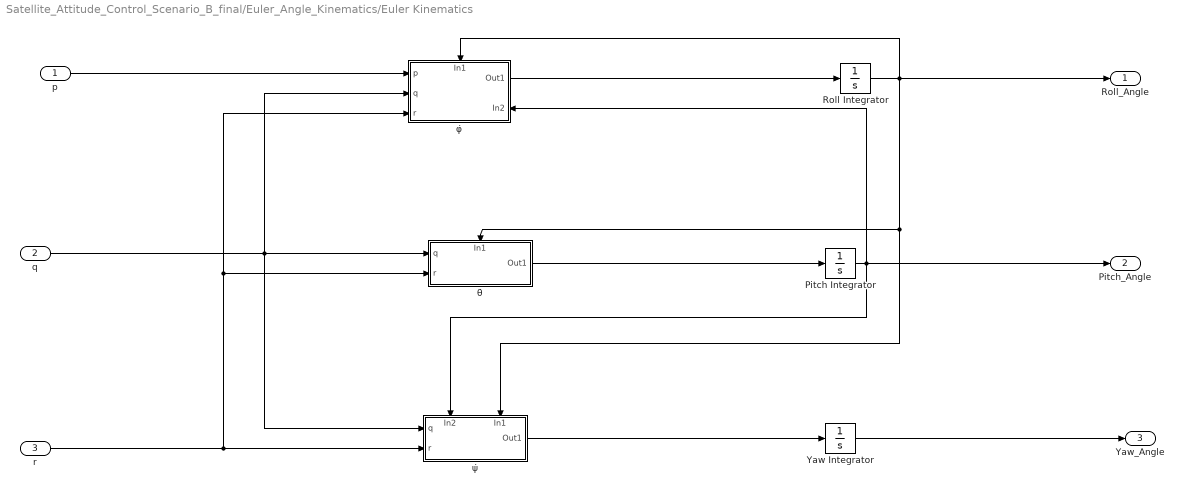
== system Satellite_Attitude_Control_Scenario_B_final/Euler_Angle_Kinematics/Euler Kinematics ==
  p : Inport
  q : Inport  Port=2
  r : Inport  Port=3
  "Pitch Integrator " : Integrator
  Roll Integrator : Integrator
  Yaw Integrator : Integrator
  θ̇ : Subsystem
      settings: PortSchema="{\"entries\":[{\"content\":{\"sides\":[{\"content\":{\"connectorIds\":[\"In1\",\"In2\"]},\"type\":\"ConnectorPlacement.EquallySpacedRectSide\",\"uuid\":\"72cd63d7-74c0-41a8-8485-738094f1ae71\"},{\"content\":{\"connectorIds\":[\"Out1\"],\"side\":\"RIGHT\"},\"type\":\"ConnectorPlacement.EquallySpacedRectSide\",\"uuid\":\"7d4a8e6a-e1d1-4310-a765-872323a4ba50\"},{\"content\":{\"connectorIds\":[\"In3\"],\"side\":\"TOP\"},\"type\":\"ConnectorPlacement.EquallySpacedRectSide\",\"uuid\":\"4f6a5b7f-2c85-44ba-8a92-ff934e310f3c\"}]},\"type\":\"ConnectorPlacement.EquallySpacedConnector\",\"uuid\":\"975b0ea9-906c-4148-abfc-d640d6ccf226\"}],\"packageUris\":[\"http://schema.mathworks.com/mf0/Connector/R2020b\"],\"version\":\"1.0\"}"
  φ̇ : Subsystem
      settings: PortSchema="{\"entries\":[{\"content\":{\"sides\":[{\"content\":{\"connectorIds\":[\"In1\",\"In2\",\"In3\"]},\"type\":\"ConnectorPlacement.EquallySpacedRectSide\",\"uuid\":\"f00c581e-14f1-4295-b4ae-0c6ffa82603e\"},{\"content\":{\"connectorIds\":[\"Out1\",\"In5\"],\"side\":\"RIGHT\"},\"type\":\"ConnectorPlacement.EquallySpacedRectSide\",\"uuid\":\"8a97a1f7-20c7-4a62-b9a7-ead15b540671\"},{\"content\":{\"connectorIds\":[\"In4\"],\"side\":\"TOP\"},\"type\":\"ConnectorPlacement.EquallySpacedRectSide\",\"uuid\":\"4686f32b-e9e5-40a1-81e7-1774be6fccb7\"},{\"content\":{\"side\":\"BOTTOM\"},\"type\":\"ConnectorPlacement.EquallySpacedRectSide\",\"uuid\":\"ecad710b-bbc0-436c-8787-a14bc0f4cb87\"}]},\"type\":\"ConnectorPlacement.EquallySpacedConnector\",\"uuid\":\"906aa43c-c71f-4267-93e4-d969eaf48c08\"}],\"packageUris\":[\"http://schema.mathworks.com/mf0/Connector/R2020b\"],\"version\":\"1.0\"}"
  ψ̇ : Subsystem
      settings: PortSchema="{\"entries\":[{\"content\":{\"sides\":[{\"content\":{\"connectorIds\":[\"In1\",\"In2\"]},\"type\":\"ConnectorPlacement.EquallySpacedRectSide\",\"uuid\":\"f2cf6a3c-1f0d-46af-9e16-2ff3fc042b92\"},{\"content\":{\"connectorIds\":[\"Out1\"],\"side\":\"RIGHT\"},\"type\":\"ConnectorPlacement.EquallySpacedRectSide\",\"uuid\":\"093aa0fc-d66f-4a39-8cfd-b4a66b9f874a\"},{\"content\":{\"connectorIds\":[\"In3\",\"In4\"],\"side\":\"TOP\"},\"type\":\"ConnectorPlacement.EquallySpacedRectSide\",\"uuid\":\"33f8a6c2-040e-4a41-a182-436f0a08e06b\"}]},\"type\":\"ConnectorPlacement.EquallySpacedConnector\",\"uuid\":\"ad1654e7-1eaa-4c9d-b0b4-793cb8860075\"}],\"packageUris\":[\"http://schema.mathworks.com/mf0/Connector/R2020b\"],\"version\":\"1.0\"}"
  Roll_Angle : Outport
  Pitch_Angle : Outport  Port=2
  Yaw_Angle : Outport  Port=3
  wires:
  p/1 -> φ̇/1(p)
  q/1 -> φ̇/2(q), ψ̇/1(q), θ̇/1(q)
  r/1 -> θ̇/2(r), φ̇/3(r), ψ̇/2(r)
  φ̇/1(Out1) -> Roll Integrator/1
  θ̇/1(Out1) -> "Pitch Integrator "/1
  ψ̇/1(Out1) -> Yaw Integrator/1
  Roll Integrator/1 -> φ̇/4(In1), Roll_Angle/1, θ̇/3(In1), ψ̇/4(In1)
  "Pitch Integrator "/1 -> Pitch_Angle/1, ψ̇/3(In2), φ̇/5(In2)
  Yaw Integrator/1 -> Yaw_Angle/1

== system Satellite_Attitude_Control_Scenario_B_final/Motor_Drive_Electronics/Current PI_X ==
  Current_Reference_X : Inport
  Measured_Current_X : Inport  Port=2
  Integrator : Integrator
  Saturation : Saturate  UpperLimit=5  LowerLimit=-5
  Sum : Sum  Inputs=|+-
  Sum1 : Sum  Inputs=|++
  integral gain : Gain  Gain=100
  proportional Gain : Gain  Gain=0.1
  Voltage_X : Outport
  wires:
  Current_Reference_X/1 -> Sum/1
  Measured_Current_X/1 -> Sum/2
  Sum/1 -> Integrator/1, proportional Gain/1
  Integrator/1 -> integral gain/1
  proportional Gain/1 -> Sum1/2
  integral gain/1 -> Sum1/1
  Sum1/1 -> Saturation/1
  Saturation/1 -> Voltage_X/1

== system Satellite_Attitude_Control_Scenario_B_final/Motor_Drive_Electronics/Current PI_Y ==
  Current_Reference_Y : Inport
  Measured_Current_Y : Inport  Port=2
  Integrator : Integrator
  Saturation : Saturate  UpperLimit=5  LowerLimit=-5
  Sum : Sum  Inputs=|+-
  Sum1 : Sum  Inputs=|++
  integral gain : Gain  Gain=100
  proportional Gain : Gain  Gain=0.1
  Voltage_Y : Outport
  wires:
  Current_Reference_Y/1 -> Sum/1
  Measured_Current_Y/1 -> Sum/2
  Sum/1 -> Integrator/1, proportional Gain/1
  Integrator/1 -> integral gain/1
  proportional Gain/1 -> Sum1/2
  integral gain/1 -> Sum1/1
  Sum1/1 -> Saturation/1
  Saturation/1 -> Voltage_Y/1

== system Satellite_Attitude_Control_Scenario_B_final/Motor_Drive_Electronics/Current PI_Z ==
  Current_Reference_Z : Inport
  Measured_Current_Z : Inport  Port=2
  Integrator : Integrator
  Saturation : Saturate  UpperLimit=5  LowerLimit=-5
  Sum : Sum  Inputs=|+-
  Sum1 : Sum  Inputs=|++
  integral gain : Gain  Gain=100
  proportional Gain : Gain  Gain=0.1
  Voltage_Z : Outport
  wires:
  Current_Reference_Z/1 -> Sum/1
  Measured_Current_Z/1 -> Sum/2
  Sum/1 -> Integrator/1, proportional Gain/1
  Integrator/1 -> integral gain/1
  proportional Gain/1 -> Sum1/2
  integral gain/1 -> Sum1/1
  Sum1/1 -> Saturation/1
  Saturation/1 -> Voltage_Z/1

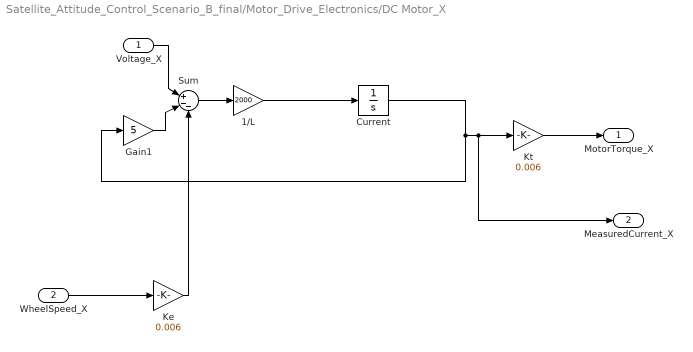
== system Satellite_Attitude_Control_Scenario_B_final/Motor_Drive_Electronics/DC Motor_X ==
  Voltage_X : Inport
  WheelSpeed_X : Inport  Port=2
  1/L : Gain  Gain=2000
  Current : Integrator
  Gain1 : Gain  Gain=5
  Ke : Gain  Gain=0.006
  Kt : Gain  Gain=0.006
  Sum : Sum  Inputs=|+--
  MotorTorque_X : Outport
  MeasuredCurrent_X : Outport  Port=2
  wires:
  1/L/1 -> Current/1
  Sum/1 -> 1/L/1
  Voltage_X/1 -> Sum/1
  Current/1 -> Gain1/1, MeasuredCurrent_X/1, Kt/1
  Kt/1 -> MotorTorque_X/1
  Gain1/1 -> Sum/2
  WheelSpeed_X/1 -> Ke/1
  Ke/1 -> Sum/3

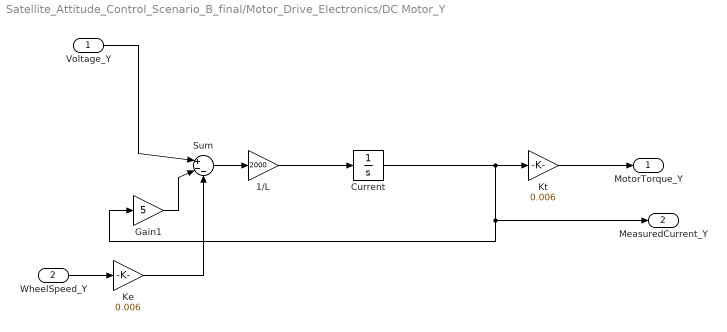
== system Satellite_Attitude_Control_Scenario_B_final/Motor_Drive_Electronics/DC Motor_Y ==
  Voltage_Y : Inport
  WheelSpeed_Y : Inport  Port=2
  1/L : Gain  Gain=2000
  Current : Integrator
  Gain1 : Gain  Gain=5
  Ke : Gain  Gain=0.006
  Kt : Gain  Gain=0.006
  Sum : Sum  Inputs=|+--
  MotorTorque_Y : Outport
  MeasuredCurrent_Y : Outport  Port=2
  wires:
  1/L/1 -> Current/1
  Sum/1 -> 1/L/1
  Voltage_Y/1 -> Sum/1
  Current/1 -> MeasuredCurrent_Y/1, Gain1/1, Kt/1
  Kt/1 -> MotorTorque_Y/1
  Gain1/1 -> Sum/2
  WheelSpeed_Y/1 -> Ke/1
  Ke/1 -> Sum/3

== system Satellite_Attitude_Control_Scenario_B_final/Motor_Drive_Electronics/DC Motor_Z ==
  Voltage_Z : Inport
  WheelSpeed_Z : Inport  Port=2
  1/L : Gain  Gain=2000
  Current : Integrator
  Gain1 : Gain  Gain=5
  Ke : Gain  Gain=0.006
  Kt : Gain  Gain=0.006
  Sum : Sum  Inputs=|+--
  MotorTorque_Z : Outport
  MeasuredCurrent_Z : Outport  Port=2
  wires:
  1/L/1 -> Current/1
  Sum/1 -> 1/L/1
  Voltage_Z/1 -> Sum/1
  Current/1 -> MeasuredCurrent_Z/1, Gain1/1, Kt/1
  Kt/1 -> MotorTorque_Z/1
  Gain1/1 -> Sum/2
  WheelSpeed_Z/1 -> Ke/1
  Ke/1 -> Sum/3

== system Satellite_Attitude_Control_Scenario_B_final/Reaction_Wheel_Dynamics/Reaction Wheel_X ==
  MotorTorque_X : Inport
  Gain : Gain  Gain=35100
  Integrator Limited : Integrator  LimitOutput=on  UpperSaturationLimit=70  LowerSaturationLimit=-70
  Sum : Sum  Inputs=|+-
  Wheel_Friction : Gain  Gain=1e-5
  ωwheel_X : Outport
  Tx : Outport  Port=2
  wires:
  Gain/1 -> Integrator Limited/1
  Sum/1 -> Gain/1
  Wheel_Friction/1 -> Sum/2
  MotorTorque_X/1 -> Tx/1, Sum/1
  Integrator Limited/1 -> ωwheel_X/1, Wheel_Friction/1

== system Satellite_Attitude_Control_Scenario_B_final/Reaction_Wheel_Dynamics/Reaction Wheel_Y ==
  MotorTorque_Y : Inport
  Gain : Gain  Gain=1/2.8490906e-5
  Integrator Limited : Integrator  LimitOutput=on  UpperSaturationLimit=70  LowerSaturationLimit=-70
  Sum : Sum  Inputs=|+-
  Wheel_Friction : Gain  Gain=1e-5
  WheelSpeed_Y : Outport
  Ty : Outport  Port=2
  wires:
  Gain/1 -> Integrator Limited/1
  Sum/1 -> Gain/1
  Wheel_Friction/1 -> Sum/2
  MotorTorque_Y/1 -> Ty/1, Sum/1
  Integrator Limited/1 -> WheelSpeed_Y/1, Wheel_Friction/1

== system Satellite_Attitude_Control_Scenario_B_final/Reaction_Wheel_Dynamics/Reaction Wheel_Z ==
  MotorTorque_Z : Inport
  Gain : Gain  Gain=1/2.8490906e-5
  Integrator Limited : Integrator  LimitOutput=on  UpperSaturationLimit=70  LowerSaturationLimit=-70
  Sum : Sum  Inputs=|+-
  Wheel_Friction : Gain  Gain=1e-5
  WheelSpeed_Z : Outport
  ReactionTorque_Z : Outport  Port=2
  wires:
  Gain/1 -> Integrator Limited/1
  Sum/1 -> Gain/1
  Wheel_Friction/1 -> Sum/2
  MotorTorque_Z/1 -> ReactionTorque_Z/1, Sum/1
  Integrator Limited/1 -> Wheel_Friction/1, WheelSpeed_Z/1

== system Satellite_Attitude_Control_Scenario_B_final/Disturbance_Torque_Summation/Disturbance_X/Aerodynamic Drag ==
  Clock : Clock
  Gain : Gain  Gain=0.03
  Gain1 : Gain  Gain=5e-8
  Trigonometric Function : Trigonometry  Operator=cos
  Out1 : Outport
  wires:
  Clock/1 -> Gain/1
  Gain/1 -> Trigonometric Function/1
  Trigonometric Function/1 -> Gain1/1
  Gain1/1 -> Out1/1

== system Satellite_Attitude_Control_Scenario_B_final/Disturbance_Torque_Summation/Disturbance_X/Gravity-Gradient ==
  Theta : Inport
  Gain : Gain  Gain=3
  Kgg : Gain  Gain=2.14e-08
  Trigonometric Function : Trigonometry
  Tdist : Outport
  wires:
  Theta/1 -> Gain/1
  Gain/1 -> Trigonometric Function/1
  Trigonometric Function/1 -> Kgg/1
  Kgg/1 -> Tdist/1

== system Satellite_Attitude_Control_Scenario_B_final/Disturbance_Torque_Summation/Disturbance_X/Solar Radiation Pressure ==
  Clock : Clock
  Gain : Gain  Gain=0.01
  Gain1 : Gain  Gain=2e-8
  Trigonometric Function : Trigonometry
  Out1 : Outport
  wires:
  Clock/1 -> Gain/1
  Gain/1 -> Trigonometric Function/1
  Trigonometric Function/1 -> Gain1/1
  Gain1/1 -> Out1/1

== system Satellite_Attitude_Control_Scenario_B_final/Disturbance_Torque_Summation/Disturbance_X/White Noise ==
  Band-Limited White Noise : simulink/Sources/Band-Limited White Noise  Cov=1  Ts=0.01  seed=[23341]
  Gain : Gain  Gain=1e-8
  Out1 : Outport
  wires:
  Band-Limited White Noise/1 -> Gain/1
  Gain/1 -> Out1/1

== system Satellite_Attitude_Control_Scenario_B_final/Disturbance_Torque_Summation/Disturbance_Y/Aerodynamic Drag ==
  Clock : Clock
  Gain : Gain  Gain=0.03
  Gain1 : Gain  Gain=5e-8
  Trigonometric Function : Trigonometry  Operator=cos
  Out1 : Outport
  wires:
  Clock/1 -> Gain/1
  Gain/1 -> Trigonometric Function/1
  Trigonometric Function/1 -> Gain1/1
  Gain1/1 -> Out1/1

== system Satellite_Attitude_Control_Scenario_B_final/Disturbance_Torque_Summation/Disturbance_Y/Gravity-Gradient ==
  Theta : Inport
  Gain : Gain  Gain=3
  Kgg : Gain  Gain=2.14e-08
  Trigonometric Function : Trigonometry
  Tdist : Outport
  wires:
  Theta/1 -> Gain/1
  Gain/1 -> Trigonometric Function/1
  Trigonometric Function/1 -> Kgg/1
  Kgg/1 -> Tdist/1

== system Satellite_Attitude_Control_Scenario_B_final/Disturbance_Torque_Summation/Disturbance_Y/Solar Radiation Pressure ==
  Clock : Clock
  Gain : Gain  Gain=0.01
  Gain1 : Gain  Gain=2e-8
  Trigonometric Function : Trigonometry
  Out1 : Outport
  wires:
  Clock/1 -> Gain/1
  Gain/1 -> Trigonometric Function/1
  Trigonometric Function/1 -> Gain1/1
  Gain1/1 -> Out1/1

== system Satellite_Attitude_Control_Scenario_B_final/Disturbance_Torque_Summation/Disturbance_Y/White Noise ==
  Band-Limited White Noise : simulink/Sources/Band-Limited White Noise  Cov=1  Ts=0.01  seed=[23341]
  Gain : Gain  Gain=1e-8
  Out1 : Outport
  wires:
  Band-Limited White Noise/1 -> Gain/1
  Gain/1 -> Out1/1

== system Satellite_Attitude_Control_Scenario_B_final/Disturbance_Torque_Summation/Disturbance_Z/Aerodynamic Drag ==
  Clock : Clock
  Gain : Gain  Gain=0.03
  Gain1 : Gain  Gain=5e-8
  Trigonometric Function : Trigonometry  Operator=cos
  Out1 : Outport
  wires:
  Clock/1 -> Gain/1
  Gain/1 -> Trigonometric Function/1
  Trigonometric Function/1 -> Gain1/1
  Gain1/1 -> Out1/1

== system Satellite_Attitude_Control_Scenario_B_final/Disturbance_Torque_Summation/Disturbance_Z/Gravity-Gradient ==
  Theta : Inport
  Gain : Gain  Gain=2
  Kgg : Gain  Gain=2.14e-08
  Trigonometric Function : Trigonometry
  Tdist : Outport
  wires:
  Theta/1 -> Gain/1
  Gain/1 -> Trigonometric Function/1
  Trigonometric Function/1 -> Kgg/1
  Kgg/1 -> Tdist/1

== system Satellite_Attitude_Control_Scenario_B_final/Disturbance_Torque_Summation/Disturbance_Z/Solar Radiation Pressure ==
  Clock : Clock
  Gain : Gain  Gain=0.01
  Gain1 : Gain  Gain=2e-8
  Trigonometric Function : Trigonometry
  Out1 : Outport
  wires:
  Clock/1 -> Gain/1
  Gain/1 -> Trigonometric Function/1
  Trigonometric Function/1 -> Gain1/1
  Gain1/1 -> Out1/1

== system Satellite_Attitude_Control_Scenario_B_final/Disturbance_Torque_Summation/Disturbance_Z/White Noise ==
  Band-Limited White Noise : simulink/Sources/Band-Limited White Noise  Cov=1  Ts=0.01  seed=[23341]
  Gain : Gain  Gain=1e-8
  Out1 : Outport
  wires:
  Band-Limited White Noise/1 -> Gain/1
  Gain/1 -> Out1/1

== system Satellite_Attitude_Control_Scenario_B_final/Euler_Angle_Kinematics/Euler Kinematics/θ̇ ==
  q : Inport
  r : Inport  Port=2
  In1 : Inport  Port=3
  Product : Product
  Product1 : Product
  Sum : Sum  Inputs=|+-
  cosϕ : Trigonometry  Operator=cos
  sinϕ : Trigonometry
  Out1 : Outport
  wires:
  q/1 -> Product/1
  cosϕ/1 -> Product/2
  r/1 -> Product1/1
  sinϕ/1 -> Product1/2
  Sum/1 -> Out1/1
  Product/1 -> Sum/1
  Product1/1 -> Sum/2
  In1/1 -> cosϕ/1, sinϕ/1

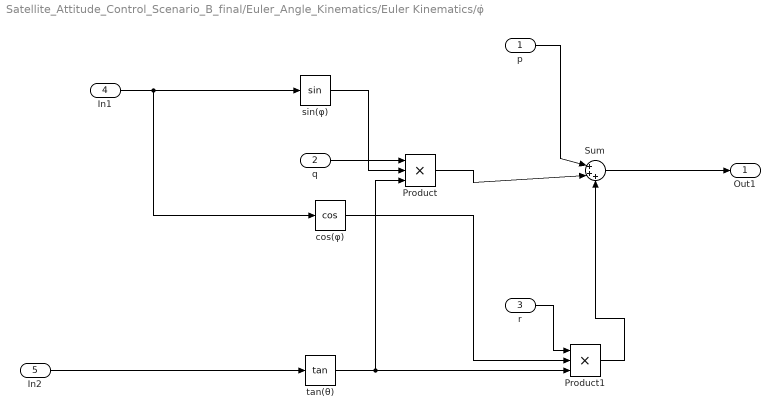
== system Satellite_Attitude_Control_Scenario_B_final/Euler_Angle_Kinematics/Euler Kinematics/φ̇ ==
  p : Inport
  q : Inport  Port=2
  r : Inport  Port=3
  In1 : Inport  Port=4
  In2 : Inport  Port=5
  Product : Product  Inputs=3
  Product1 : Product  Inputs=3
  Sum : Sum  Inputs=|+++
  "cos(φ) " : Trigonometry  Operator=cos
  "sin(φ) " : Trigonometry
  "tan(θ) " : Trigonometry  Operator=tan
  Out1 : Outport
  wires:
  q/1 -> Product/1
  "sin(φ) "/1 -> Product/2
  "tan(θ) "/1 -> Product1/3, Product/3
  p/1 -> Sum/1
  Product/1 -> Sum/2
  r/1 -> Product1/1
  "cos(φ) "/1 -> Product1/2
  Product1/1 -> Sum/3
  Sum/1 -> Out1/1
  In2/1 -> "tan(θ) "/1
  In1/1 -> "cos(φ) "/1, "sin(φ) "/1

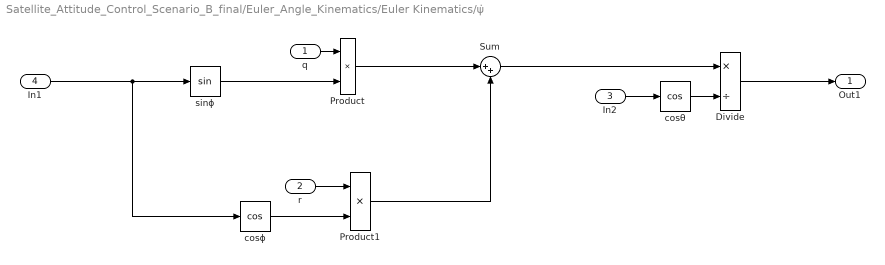
== system Satellite_Attitude_Control_Scenario_B_final/Euler_Angle_Kinematics/Euler Kinematics/ψ̇ ==
  q : Inport
  r : Inport  Port=2
  In2 : Inport  Port=3
  In1 : Inport  Port=4
  Divide : Product  Inputs=*/
  Product : Product
  Product1 : Product
  Sum : Sum  Inputs=|++
  cosθ : Trigonometry  Operator=cos
  cosϕ : Trigonometry  Operator=cos
  sinϕ : Trigonometry
  Out1 : Outport
  wires:
  q/1 -> Product/1
  sinϕ/1 -> Product/2
  r/1 -> Product1/1
  cosϕ/1 -> Product1/2
  Product/1 -> Sum/1
  Product1/1 -> Sum/2
  Sum/1 -> Divide/1
  cosθ/1 -> Divide/2
  Divide/1 -> Out1/1
  In2/1 -> cosθ/1
  In1/1 -> cosϕ/1, sinϕ/1
